simulink model "voltage_to_speed_m_per_s"  (R2020b)
settings: Solver=VariableStepAuto  StartTime=0.0  StopTime=10.0  RelTol=1e-3
settings Model: Creator=Training  LastModifiedBy=Training

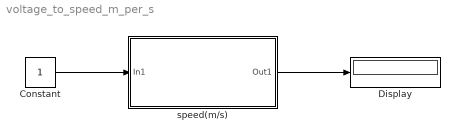
== system voltage_to_speed_m_per_s ==
  Constant : Constant
  Display : Display
  speed(m/s) : Subsystem
  wires:
  Constant/1 -> speed(m/s)/1(In1)
  speed(m/s)/1(Out1) -> Display/1

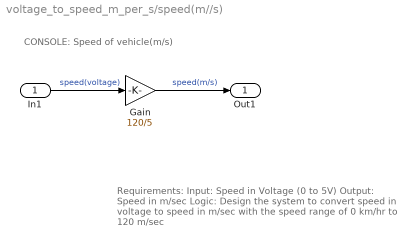
== system voltage_to_speed_m_per_s/speed(m//s) ==
  note: CONSOLE: Speed of vehicle(m/s)
  note: Requirements:
      | Input: Speed in Voltage (0 to 5V)
      | Output: Speed in m/sec
      | Logic: Design the system to convert speed in voltage to
      | speed in m/sec with the speed range of 0 km/hr to 120 m/sec
  In1 : Inport
  Gain : Gain  Gain=120/5
  Out1 : Outport
  wires:
  In1/1 -> Gain/1  "speed(voltage)"
  Gain/1 -> Out1/1  "speed(m/s)"
